simulink model "CanardUAV_Flight_Control_Using_PID"  (R2020b)
settings: Solver=VariableStepAuto  StartTime=0  StopTime=30  FixedStep=1e-4  MaxStep=1e-2  RelTol=1e-3
libraries: slpidlib x6
settings Model: Creator=Adisu  LastModifiedBy=ysDeng
settings DataIOCC: SaveFormat=StructureWithTime  ReturnWorkspaceOutputs=off
settings OptimizationCC: BlockReduction=off  BufferReuse=off
settings DebuggingCC: AlgebraicLoopMsg=none  UnconnectedInputMsg=none  UnconnectedOutputMsg=none  UnconnectedLineMsg=none

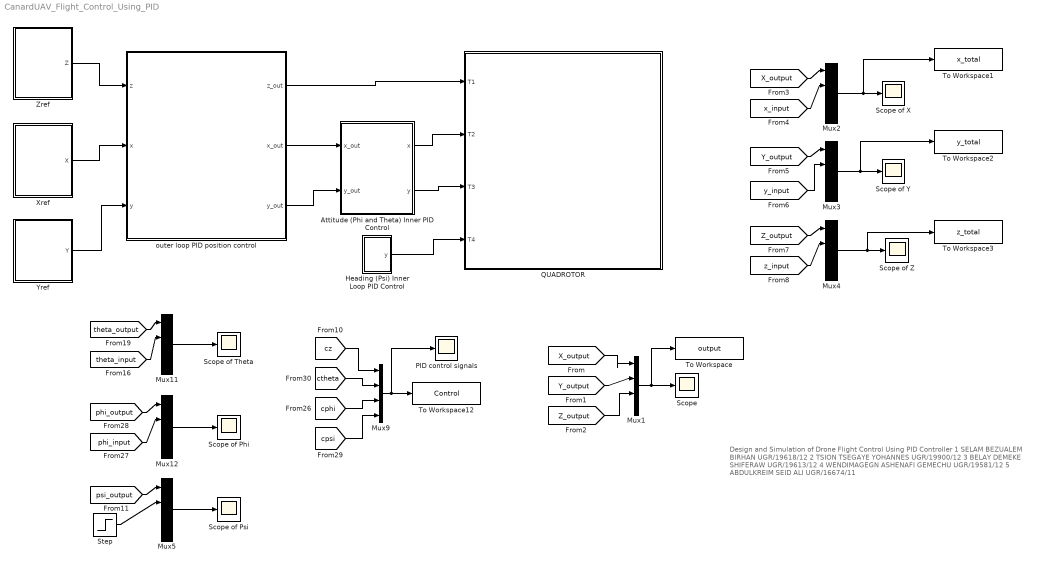
== system CanardUAV_Flight_Control_Using_PID ==
  note: Design and Simulation of Drone Flight Control Using PID Controller
      |
      | 1 SELAM BEZUALEM BIRHAN UGR/19618/12
      | 2 TSION TSEGAYE YOHANNES UGR/19900/12
      | 3 BELAY DEMEKE SHIFERAW UGR/19613/12
      | 4 WENDIMAGEGN ASHENAFI GEMECHU UGR/19581/12
      | 5 ABDULKREIM SEID ALI UGR/16674/11
  Attitude (Phi and Theta) Inner PID Control : Subsystem
  Heading (Psi) Inner Loop PID Control : Subsystem
  Mux1 : Mux  Inputs=3
  Mux{2..5,11..12} (6 alike) : Mux  Inputs=2
  Mux9 : Mux
  PID control signals : Scope
  "QUADROTOR " : Subsystem
      mask Display: image('$imagefile'); % Use "Edit Image" on toolstrip to change.
  Scope : Scope
  Scope of Phi : Scope
  Scope of Psi : Scope
  Scope of Theta : Scope
  Scope of X : Scope
  Scope of Y : Scope
  Scope of Z : Scope
  Step : Step  Time=5  After=0.2  SampleTime=0
  To Workspace : ToWorkspace  VariableName=output  SaveFormat=Timeseries  SampleTime=-1
  To Workspace1 : ToWorkspace  VariableName=x_total  SaveFormat=Timeseries  SampleTime=-1
  To Workspace12 : ToWorkspace  VariableName=Control  SampleTime=-1
      settings: Save2DSignal=2-D array (concatenate along first dimension)
  To Workspace2 : ToWorkspace  VariableName=y_total  SaveFormat=Timeseries  SampleTime=-1
  To Workspace3 : ToWorkspace  VariableName=z_total  SaveFormat=Timeseries  SampleTime=-1
  Xref : Subsystem
      mask Display: image('C:\Users\Mo\Desktop\Porject files\Mathlab\9KgUe.png'); % Use "Edit Image" on toolstrip to change.
  Yref : Subsystem
      mask Display: image('$imagefile'); % Use "Edit Image" on toolstrip to change.
  Zref : Subsystem
      mask Display: image('C:\Users\Mo\Desktop\Porject files\Mathlab\9KgUe.png'); % Use "Edit Image" on toolstrip to change.
  outer loop PID position control : Subsystem
  wires:
  Attitude (Phi and Theta) Inner PID Control/2(y) -> "QUADROTOR "/3(T3)
  outer loop PID position control/3(y_out) -> Attitude (Phi and Theta) Inner PID Control/2(y_out)
  outer loop PID position control/2(x_out) -> Attitude (Phi and Theta) Inner PID Control/1(x_out)
  outer loop PID position control/1(z_out) -> "QUADROTOR "/1(T1)
  Heading (Psi) Inner Loop PID Control/1(y) -> "QUADROTOR "/4(T4)
  Attitude (Phi and Theta) Inner PID Control/1(x) -> "QUADROTOR "/2(T2)
  [theta_input] -> Mux11/2
  Mux11/1 -> Scope of Theta/1
  [theta_output] -> Mux11/1
  [phi_input] -> Mux12/2
  Mux12/1 -> Scope of Phi/1
  [phi_output] -> Mux12/1
  Mux9/1 -> PID control signals/1, To Workspace12/1
  [cz] -> Mux9/1
  Zref/1(Z) -> outer loop PID position control/1(z)
  Xref/1(X) -> outer loop PID position control/2(x)
  Yref/1(Y) -> outer loop PID position control/3(y)
  [X_output] -> Mux1/1
  [Y_output] -> Mux1/2
  [Z_output] -> Mux1/3
  Mux1/1 -> To Workspace/1, Scope/1
  [X_output] -> Mux2/1
  [x_input] -> Mux2/2
  Mux2/1 -> To Workspace1/1, Scope of X/1
  Mux3/1 -> To Workspace2/1, Scope of Y/1
  [y_input] -> Mux3/2
  [Y_output] -> Mux3/1
  [Z_output] -> Mux4/1
  [z_input] -> Mux4/2
  Mux4/1 -> To Workspace3/1, Scope of Z/1
  [psi_output] -> Mux5/1
  Mux5/1 -> Scope of Psi/1
  Step/1 -> Mux5/2
  [ctheta] -> Mux9/2
  [cphi] -> Mux9/3
  [cpsi] -> Mux9/4

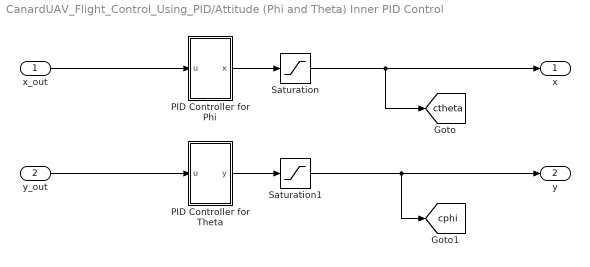
== system CanardUAV_Flight_Control_Using_PID/Attitude (Phi and Theta) Inner PID Control ==
  x_out : Inport
  y_out : Inport  Port=2
  PID Controller for Phi : Subsystem
  PID Controller for Theta : Subsystem
  Saturation : Saturate  UpperLimit=1  LowerLimit=-1
  Saturation1 : Saturate  UpperLimit=1  LowerLimit=-1
  x : Outport
  y : Outport  Port=2
  tag scope: cphi=global, ctheta=global
  wires:
  PID Controller for Phi/1(x) -> Saturation/1
  x_out/1 -> PID Controller for Phi/1(u)
  PID Controller for Theta/1(y) -> Saturation1/1
  Saturation1/1 -> [cphi], y/1
  Saturation/1 -> x/1, [ctheta]
  y_out/1 -> PID Controller for Theta/1(u)

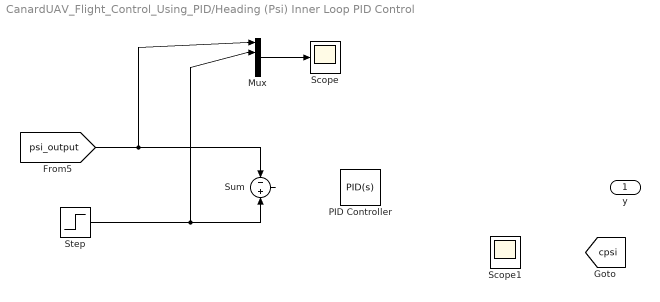
== system CanardUAV_Flight_Control_Using_PID/Heading (Psi) Inner Loop PID Control ==
  Mux : Mux  Inputs=2
  PID Controller : slpidlib/PID Controller  Controller=PID  Form=Parallel  TimeDomain=Continuous-time  UseExternalTs=off  SampleTime=-1  IntegratorMethod=Forward Euler  FilterMethod=Forward Euler  ControllerParametersSource=internal  P=0.000984100095340088  I=4.60704277684503e-05  UseKiTs=off  D=0.00516178120248641  N=5.45397025421619  UseFilter=on  TunerSelectOption=Transfer Function Based (PID Tuner App)  InitialConditionSource=internal  InitialConditionForIntegrator=0  InitialConditionForFilter=0  DifferentiatorICPrevScaledInput=0  ExternalReset=none  TrackingMode=off  Kt=1  LimitOutput=off  SatLimitsSource=internal  UpperSaturationLimit=inf  LowerSaturationLimit=-inf  LinearizeAsGain=on  AntiWindupMode=none  Kb=1  LimitIntegrator=off  UpperIntegratorSaturationLimit=inf  LowerIntegratorSaturationLimit=-inf  POutMin=[]  POutMax=[]  IOutMin=[]  IOutMax=[]  DOutMin=[]  DOutMax=[]  NOutMin=[]  NOutMax=[]  SumOutMin=[]  SumOutMax=[]  SaturationOutMin=[]  SaturationOutMax=[]  PParamMin=[]  PParamMax=[]  IParamMin=[]  IParamMax=[]  DParamMin=[]  DParamMax=[]  NParamMin=[]  NParamMax=[]  KbParamMin=[]  KbParamMax=[]  KtParamMin=[]  KtParamMax=[]  KbOutMin=[]  KbOutMax=[]  KtOutMin=[]  KtOutMax=[]  IntegratorOutMin=[]  IntegratorOutMax=[]  FilterOutMin=[]  FilterOutMax=[]  SumI1OutMin=[]  SumI1OutMax=[]  SumI2OutMin=[]  SumI2OutMax=[]  SumI3OutMin=[]  SumI3OutMax=[]  SumI4OutMin=[]  SumI4OutMax=[]  SumDOutMin=[]  SumDOutMax=[]  DifferentiatorOutMin=[]  DifferentiatorOutMax=[]  FilterDiffOutCoefMin=[]  FilterDiffOutCoefMax=[]  ReciprocalOutMin=[]  ReciprocalOutMax=[]  SumDenOutMin=[]  SumDenOutMax=[]  SumNumOutMin=[]  SumNumOutMax=[]  DivideOutMin=[]  DivideOutMax=[]  UdiffTsProdOutMin=[]  UdiffTsProdOutMax=[]  NTsProdOutMin=[]  NTsProdOutMax=[]  UintegralTsProdOutMin=[]  UintegralTsProdOutMax=[]  UngainTsProdOutMin=[]  UngainTsProdOutMax=[]  ClampingZeroOutDataTypeStr=Inherit: Inherit via back propagation  ClampingZeroOutMin=[]  ClampingZeroOutMax=[]  FilterDenConstantOutDataTypeStr=Inherit: Inherit via back propagation  FilterDenConstantOutMin=[]  FilterDenConstantOutMax=[]  PCopyOutDataTypeStr=Inherit: Inherit via back propagation  PCopyOutMin=[]  PCopyOutMax=[]  NCopyOutDataTypeStr=Inherit: Inherit via back propagation  NCopyOutMin=[]  NCopyOutMax=[]  IntegratorContinuousStateAttributes=''  IntegratorStateMustResolveToSignalObject=off  IntegratorRTWStateStorageClass=Auto  FilterContinuousStateAttributes=''  FilterStateMustResolveToSignalObject=off  FilterRTWStateStorageClass=Auto  ParallelPVariant=InternalParameters  IdealPVariant=Disabled  IVariant=InternalParameters  DVariant=InternalParameters  IntegratorVariant=Continuous  SatVariant=Disabled  AWVariant=Passthrough  PCopyVariant=Disabled  TRVariant=Disabled  FdbkBlocksVariant=Forward  IdealPFdbkVariant=Disabled  SatFdbkVariant=Disabled  DerivativeFilterVariant=ContFilter  NVariant=InternalParameters  NCopyVariant=Disabled  FilterICVariant=InternalICsFilter  IntegratorICVariant=InternalICs  ExternalResetVariant=Disabled  TRSumVariant=Passthrough  SumFdbkVariant=Disabled  SumVariant=Sum_PID  TsampFilterVariant=InternalTs  TsampNgainVariant=Passthrough  TsampIntegralVariant=Disabled_SignalSpec  ExternalSaturationOutDataTypeStr=Inherit: Same as second input
  Scope : Scope
  Scope1 : Scope
  Step : Step  Time=5  After=0.2  SampleTime=0
  Sum : Sum  Inputs=-+
  y : Outport
  tag scope: cpsi=global
  wires:
  [psi_output] -> Mux/1, Sum/1
  Sum/1 -> ?
  Mux/1 -> Scope/1
  ? -> y/1, [cpsi], Scope1/1
  Step/1 -> Sum/2, Mux/2

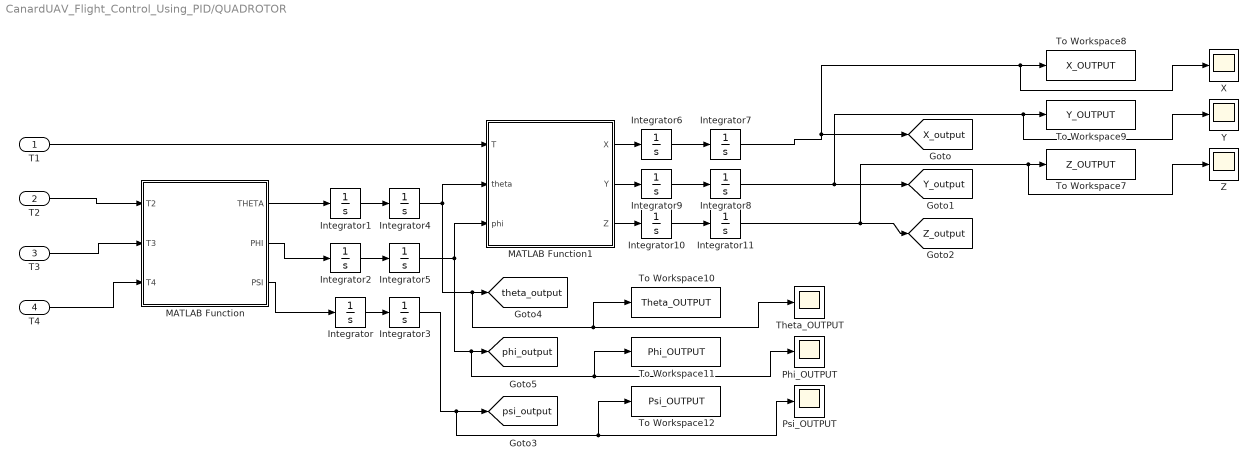
== system CanardUAV_Flight_Control_Using_PID/QUADROTOR  ==
  T1 : Inport
  T2 : Inport  Port=2
  T3 : Inport  Port=3
  T4 : Inport  Port=4
  Integrator{,1..11} (12 alike) : Integrator
  MATLAB Function : MATLAB Function  TreatAsAtomicUnit=on
  MATLAB Function1 : MATLAB Function  TreatAsAtomicUnit=on
  Phi_OUTPUT : Scope
  Psi_OUTPUT : Scope
  Theta_OUTPUT : Scope
  To Workspace10 : ToWorkspace  VariableName=Theta_OUTPUT  SampleTime=-1
      settings: Save2DSignal=2-D array (concatenate along first dimension)
  To Workspace11 : ToWorkspace  VariableName=Phi_OUTPUT  SampleTime=-1
      settings: Save2DSignal=2-D array (concatenate along first dimension)
  To Workspace12 : ToWorkspace  VariableName=Psi_OUTPUT  SampleTime=-1
      settings: Save2DSignal=2-D array (concatenate along first dimension)
  To Workspace7 : ToWorkspace  VariableName=Z_OUTPUT  SampleTime=-1
      settings: Save2DSignal=2-D array (concatenate along first dimension)
  To Workspace8 : ToWorkspace  VariableName=X_OUTPUT  SampleTime=-1
      settings: Save2DSignal=2-D array (concatenate along first dimension)
  To Workspace9 : ToWorkspace  VariableName=Y_OUTPUT  SampleTime=-1
      settings: Save2DSignal=2-D array (concatenate along first dimension)
  X : Scope
  Y : Scope
  Z : Scope
  tag scope: X_output=global, Y_output=global, Z_output=global, phi_output=global, psi_output=global, theta_output=global
  wires:
  MATLAB Function/3(PSI) -> Integrator/1
  Integrator9/1 -> Integrator8/1
  Integrator10/1 -> Integrator11/1
  Integrator6/1 -> Integrator7/1
  Integrator1/1 -> Integrator4/1
  MATLAB Function1/2(Y) -> Integrator9/1
  Integrator2/1 -> Integrator5/1
  MATLAB Function1/1(X) -> Integrator6/1
  MATLAB Function1/3(Z) -> Integrator10/1
  Integrator/1 -> Integrator3/1
  MATLAB Function/1(THETA) -> Integrator1/1
  T2/1 -> MATLAB Function/1(T2)
  MATLAB Function/2(PHI) -> Integrator2/1
  Integrator8/1 -> Y/1, To Workspace9/1, [Y_output]
  Integrator4/1 -> To Workspace10/1, Theta_OUTPUT/1, [theta_output], MATLAB Function1/2(theta)
  T1/1 -> MATLAB Function1/1(T)
  Integrator5/1 -> To Workspace11/1, Phi_OUTPUT/1, [phi_output], MATLAB Function1/3(phi)
  T3/1 -> MATLAB Function/2(T3)
  Integrator11/1 -> Z/1, To Workspace7/1, [Z_output]
  T4/1 -> MATLAB Function/3(T4)
  Integrator3/1 -> Psi_OUTPUT/1, To Workspace12/1, [psi_output]
  Integrator7/1 -> X/1, To Workspace8/1, [X_output]

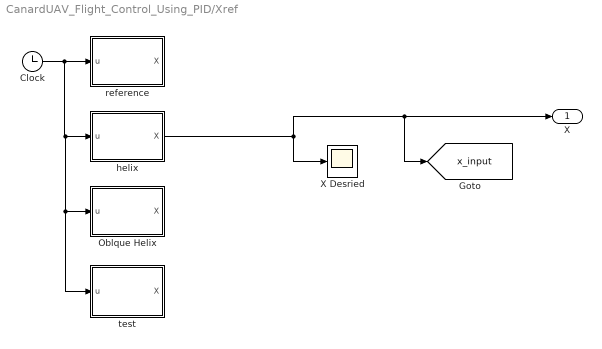
== system CanardUAV_Flight_Control_Using_PID/Xref ==
  Clock : Clock
      settings: Decimation=200
  Oblque Helix : MATLAB Function  TreatAsAtomicUnit=on
  X Desried : Scope
  helix : MATLAB Function  TreatAsAtomicUnit=on
  reference : MATLAB Function  TreatAsAtomicUnit=on
  test : MATLAB Function  TreatAsAtomicUnit=on
  X : Outport
  tag scope: x_input=global
  wires:
  helix/1(X) -> X Desried/1, [x_input], X/1
  Clock/1 -> test/1(u), Oblque Helix/1(u), helix/1(u), reference/1(u)

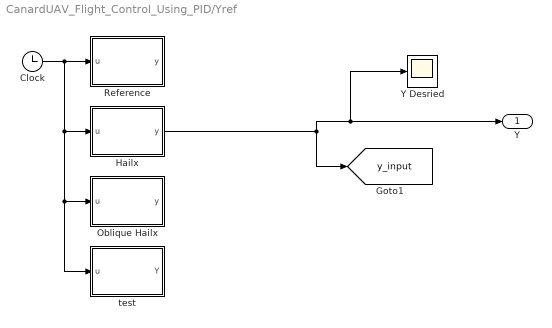
== system CanardUAV_Flight_Control_Using_PID/Yref ==
  Clock : Clock
      settings: Decimation=200
  Hailx : MATLAB Function  TreatAsAtomicUnit=on
  Oblique Hailx : MATLAB Function  TreatAsAtomicUnit=on
  Reference : MATLAB Function  TreatAsAtomicUnit=on
  Y Desried : Scope
  test : MATLAB Function  TreatAsAtomicUnit=on
  Y : Outport
  tag scope: y_input=global
  wires:
  Hailx/1(y) -> [y_input], Y Desried/1, Y/1
  Clock/1 -> test/1(u), Oblique Hailx/1(u), Hailx/1(u), Reference/1(u)

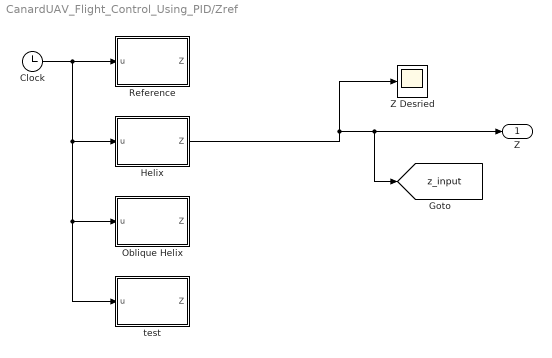
== system CanardUAV_Flight_Control_Using_PID/Zref ==
  Clock : Clock
      settings: Decimation=200
  Helix : MATLAB Function  TreatAsAtomicUnit=on
  Oblique Helix : MATLAB Function  TreatAsAtomicUnit=on
  Reference : MATLAB Function  TreatAsAtomicUnit=on
  Z Desried : Scope
  test : MATLAB Function  TreatAsAtomicUnit=on
  Z : Outport
  tag scope: z_input=global
  wires:
  Helix/1(Z) -> Z Desried/1, [z_input], Z/1
  Clock/1 -> Reference/1(u), Helix/1(u), test/1(u), Oblique Helix/1(u)

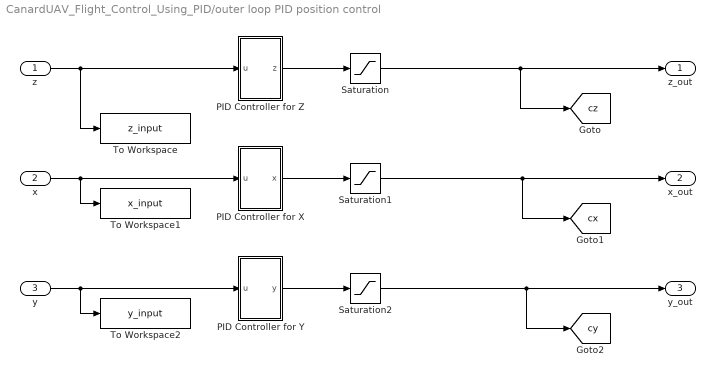
== system CanardUAV_Flight_Control_Using_PID/outer loop PID position control ==
  z : Inport
  x : Inport  Port=2
  y : Inport  Port=3
  PID Controller for X : Subsystem
  PID Controller for Y : Subsystem
  PID Controller for Z : Subsystem
  Saturation : Saturate  UpperLimit=8  LowerLimit=0
  Saturation1 : Saturate  UpperLimit=1  LowerLimit=-1
  Saturation2 : Saturate  UpperLimit=1  LowerLimit=-1
  To Workspace : ToWorkspace  VariableName=z_input  SaveFormat=Timeseries  SampleTime=-1
  To Workspace1 : ToWorkspace  VariableName=x_input  SaveFormat=Timeseries  SampleTime=-1
  To Workspace2 : ToWorkspace  VariableName=y_input  SaveFormat=Timeseries  SampleTime=-1
  z_out : Outport
  x_out : Outport  Port=2
  y_out : Outport  Port=3
  tag scope: cx=global, cy=global, cz=global
  wires:
  PID Controller for Z/1(z) -> Saturation/1
  PID Controller for Y/1(y) -> Saturation2/1
  PID Controller for X/1(x) -> Saturation1/1
  z/1 -> To Workspace/1, PID Controller for Z/1(u)
  Saturation/1 -> [cz], z_out/1
  Saturation1/1 -> x_out/1, [cx]
  Saturation2/1 -> y_out/1, [cy]
  x/1 -> To Workspace1/1, PID Controller for X/1(u)
  y/1 -> To Workspace2/1, PID Controller for Y/1(u)

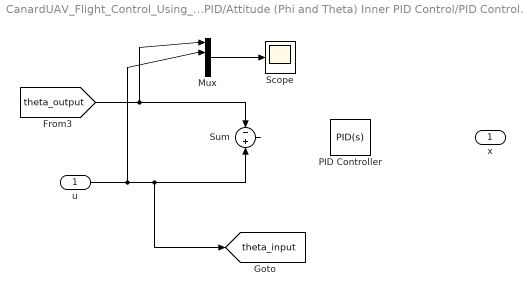
== system CanardUAV_Flight_Control_Using_PID/Attitude (Phi and Theta) Inner PID Control/PID Controller for Phi ==
  u : Inport
  Mux : Mux  Inputs=2
  PID Controller : slpidlib/PID Controller  Controller=PID  Form=Parallel  TimeDomain=Continuous-time  UseExternalTs=off  SampleTime=-1  IntegratorMethod=Forward Euler  FilterMethod=Forward Euler  ControllerParametersSource=internal  P=1.9891252123158  I=5.9601995006883  UseKiTs=off  D=0.159826669701916  N=399.033800628707  UseFilter=on  TunerSelectOption=Transfer Function Based (PID Tuner App)  InitialConditionSource=internal  InitialConditionForIntegrator=0  InitialConditionForFilter=0  DifferentiatorICPrevScaledInput=0  ExternalReset=none  TrackingMode=off  Kt=1  LimitOutput=off  SatLimitsSource=internal  UpperSaturationLimit=inf  LowerSaturationLimit=-inf  LinearizeAsGain=on  AntiWindupMode=none  Kb=1  LimitIntegrator=off  UpperIntegratorSaturationLimit=inf  LowerIntegratorSaturationLimit=-inf  POutMin=[]  POutMax=[]  IOutMin=[]  IOutMax=[]  DOutMin=[]  DOutMax=[]  NOutMin=[]  NOutMax=[]  SumOutMin=[]  SumOutMax=[]  SaturationOutMin=[]  SaturationOutMax=[]  PParamMin=[]  PParamMax=[]  IParamMin=[]  IParamMax=[]  DParamMin=[]  DParamMax=[]  NParamMin=[]  NParamMax=[]  KbParamMin=[]  KbParamMax=[]  KtParamMin=[]  KtParamMax=[]  KbOutMin=[]  KbOutMax=[]  KtOutMin=[]  KtOutMax=[]  IntegratorOutMin=[]  IntegratorOutMax=[]  FilterOutMin=[]  FilterOutMax=[]  SumI1OutMin=[]  SumI1OutMax=[]  SumI2OutMin=[]  SumI2OutMax=[]  SumI3OutMin=[]  SumI3OutMax=[]  SumI4OutMin=[]  SumI4OutMax=[]  SumDOutMin=[]  SumDOutMax=[]  DifferentiatorOutMin=[]  DifferentiatorOutMax=[]  FilterDiffOutCoefMin=[]  FilterDiffOutCoefMax=[]  ReciprocalOutMin=[]  ReciprocalOutMax=[]  SumDenOutMin=[]  SumDenOutMax=[]  SumNumOutMin=[]  SumNumOutMax=[]  DivideOutMin=[]  DivideOutMax=[]  UdiffTsProdOutMin=[]  UdiffTsProdOutMax=[]  NTsProdOutMin=[]  NTsProdOutMax=[]  UintegralTsProdOutMin=[]  UintegralTsProdOutMax=[]  UngainTsProdOutMin=[]  UngainTsProdOutMax=[]  ClampingZeroOutDataTypeStr=Inherit: Inherit via back propagation  ClampingZeroOutMin=[]  ClampingZeroOutMax=[]  FilterDenConstantOutDataTypeStr=Inherit: Inherit via back propagation  FilterDenConstantOutMin=[]  FilterDenConstantOutMax=[]  PCopyOutDataTypeStr=Inherit: Inherit via back propagation  PCopyOutMin=[]  PCopyOutMax=[]  NCopyOutDataTypeStr=Inherit: Inherit via back propagation  NCopyOutMin=[]  NCopyOutMax=[]  IntegratorContinuousStateAttributes=''  IntegratorStateMustResolveToSignalObject=off  IntegratorRTWStateStorageClass=Auto  FilterContinuousStateAttributes=''  FilterStateMustResolveToSignalObject=off  FilterRTWStateStorageClass=Auto  ParallelPVariant=InternalParameters  IdealPVariant=Disabled  IVariant=InternalParameters  DVariant=InternalParameters  IntegratorVariant=Continuous  SatVariant=Disabled  AWVariant=Passthrough  PCopyVariant=Disabled  TRVariant=Disabled  FdbkBlocksVariant=Forward  IdealPFdbkVariant=Disabled  SatFdbkVariant=Disabled  DerivativeFilterVariant=ContFilter  NVariant=InternalParameters  NCopyVariant=Disabled  FilterICVariant=InternalICsFilter  IntegratorICVariant=InternalICs  ExternalResetVariant=Disabled  TRSumVariant=Passthrough  SumFdbkVariant=Disabled  SumVariant=Sum_PID  TsampFilterVariant=InternalTs  TsampNgainVariant=Passthrough  TsampIntegralVariant=Disabled_SignalSpec  ExternalSaturationOutDataTypeStr=Inherit: Same as second input
  Scope : Scope
  Sum : Sum  Inputs=-+
  x : Outport
  tag scope: theta_input=global
  wires:
  [theta_output] -> Mux/1, Sum/1
  u/1 -> Mux/2, [theta_input], Sum/2
  Sum/1 -> ?
  Mux/1 -> Scope/1
  ? -> x/1

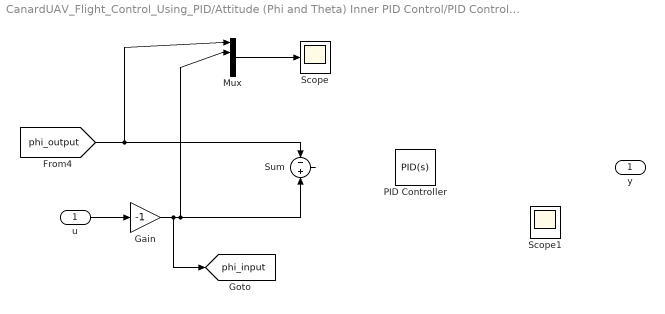
== system CanardUAV_Flight_Control_Using_PID/Attitude (Phi and Theta) Inner PID Control/PID Controller for Theta ==
  u : Inport
  Gain : Gain  Gain=-1
  Mux : Mux  Inputs=2
  PID Controller : slpidlib/PID Controller  Controller=PID  Form=Parallel  TimeDomain=Continuous-time  UseExternalTs=off  SampleTime=-1  IntegratorMethod=Forward Euler  FilterMethod=Forward Euler  ControllerParametersSource=internal  P=0.0999  I=0.01  UseKiTs=off  D=0.22  N=100  UseFilter=on  TunerSelectOption=Transfer Function Based (PID Tuner App)  InitialConditionSource=internal  InitialConditionForIntegrator=0  InitialConditionForFilter=0  DifferentiatorICPrevScaledInput=0  ExternalReset=none  TrackingMode=off  Kt=1  LimitOutput=off  SatLimitsSource=internal  UpperSaturationLimit=inf  LowerSaturationLimit=-inf  LinearizeAsGain=on  AntiWindupMode=none  Kb=1  LimitIntegrator=off  UpperIntegratorSaturationLimit=inf  LowerIntegratorSaturationLimit=-inf  POutMin=[]  POutMax=[]  IOutMin=[]  IOutMax=[]  DOutMin=[]  DOutMax=[]  NOutMin=[]  NOutMax=[]  SumOutMin=[]  SumOutMax=[]  SaturationOutMin=[]  SaturationOutMax=[]  PParamMin=[]  PParamMax=[]  IParamMin=[]  IParamMax=[]  DParamMin=[]  DParamMax=[]  NParamMin=[]  NParamMax=[]  KbParamMin=[]  KbParamMax=[]  KtParamMin=[]  KtParamMax=[]  KbOutMin=[]  KbOutMax=[]  KtOutMin=[]  KtOutMax=[]  IntegratorOutMin=[]  IntegratorOutMax=[]  FilterOutMin=[]  FilterOutMax=[]  SumI1OutMin=[]  SumI1OutMax=[]  SumI2OutMin=[]  SumI2OutMax=[]  SumI3OutMin=[]  SumI3OutMax=[]  SumI4OutMin=[]  SumI4OutMax=[]  SumDOutMin=[]  SumDOutMax=[]  DifferentiatorOutMin=[]  DifferentiatorOutMax=[]  FilterDiffOutCoefMin=[]  FilterDiffOutCoefMax=[]  ReciprocalOutMin=[]  ReciprocalOutMax=[]  SumDenOutMin=[]  SumDenOutMax=[]  SumNumOutMin=[]  SumNumOutMax=[]  DivideOutMin=[]  DivideOutMax=[]  UdiffTsProdOutMin=[]  UdiffTsProdOutMax=[]  NTsProdOutMin=[]  NTsProdOutMax=[]  UintegralTsProdOutMin=[]  UintegralTsProdOutMax=[]  UngainTsProdOutMin=[]  UngainTsProdOutMax=[]  ClampingZeroOutDataTypeStr=Inherit: Inherit via back propagation  ClampingZeroOutMin=[]  ClampingZeroOutMax=[]  FilterDenConstantOutDataTypeStr=Inherit: Inherit via back propagation  FilterDenConstantOutMin=[]  FilterDenConstantOutMax=[]  PCopyOutDataTypeStr=Inherit: Inherit via back propagation  PCopyOutMin=[]  PCopyOutMax=[]  NCopyOutDataTypeStr=Inherit: Inherit via back propagation  NCopyOutMin=[]  NCopyOutMax=[]  IntegratorContinuousStateAttributes=''  IntegratorStateMustResolveToSignalObject=off  IntegratorRTWStateStorageClass=Auto  FilterContinuousStateAttributes=''  FilterStateMustResolveToSignalObject=off  FilterRTWStateStorageClass=Auto  ParallelPVariant=InternalParameters  IdealPVariant=Disabled  IVariant=InternalParameters  DVariant=InternalParameters  IntegratorVariant=Continuous  SatVariant=Disabled  AWVariant=Passthrough  PCopyVariant=Disabled  TRVariant=Disabled  FdbkBlocksVariant=Forward  IdealPFdbkVariant=Disabled  SatFdbkVariant=Disabled  DerivativeFilterVariant=ContFilter  NVariant=InternalParameters  NCopyVariant=Disabled  FilterICVariant=InternalICsFilter  IntegratorICVariant=InternalICs  ExternalResetVariant=Disabled  TRSumVariant=Passthrough  SumFdbkVariant=Disabled  SumVariant=Sum_PID  TsampFilterVariant=InternalTs  TsampNgainVariant=Passthrough  TsampIntegralVariant=Disabled_SignalSpec  ExternalSaturationOutDataTypeStr=Inherit: Same as second input
  Scope : Scope
  Scope1 : Scope
  Sum : Sum  Inputs=-+
  y : Outport
  tag scope: phi_input=global
  wires:
  [phi_output] -> Mux/1, Sum/1
  Mux/1 -> Scope/1
  Sum/1 -> ?
  u/1 -> Gain/1
  Gain/1 -> [phi_input], Mux/2, Sum/2
  ? -> y/1, Scope1/1

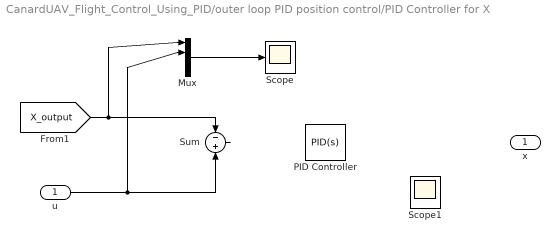
== system CanardUAV_Flight_Control_Using_PID/outer loop PID position control/PID Controller for X ==
  u : Inport
  Mux : Mux  Inputs=2
  PID Controller : slpidlib/PID Controller  Controller=PID  Form=Parallel  TimeDomain=Continuous-time  UseExternalTs=off  SampleTime=-1  IntegratorMethod=Forward Euler  FilterMethod=Forward Euler  ControllerParametersSource=internal  P=0.0999  I=0.031  UseKiTs=off  D=0.22  N=100  UseFilter=on  TunerSelectOption=Transfer Function Based (PID Tuner App)  InitialConditionSource=internal  InitialConditionForIntegrator=0  InitialConditionForFilter=0  DifferentiatorICPrevScaledInput=0  ExternalReset=none  TrackingMode=off  Kt=1  LimitOutput=off  SatLimitsSource=internal  UpperSaturationLimit=inf  LowerSaturationLimit=-inf  LinearizeAsGain=on  AntiWindupMode=none  Kb=1  LimitIntegrator=off  UpperIntegratorSaturationLimit=inf  LowerIntegratorSaturationLimit=-inf  POutMin=[]  POutMax=[]  IOutMin=[]  IOutMax=[]  DOutMin=[]  DOutMax=[]  NOutMin=[]  NOutMax=[]  SumOutMin=[]  SumOutMax=[]  SaturationOutMin=[]  SaturationOutMax=[]  PParamMin=[]  PParamMax=[]  IParamMin=[]  IParamMax=[]  DParamMin=[]  DParamMax=[]  NParamMin=[]  NParamMax=[]  KbParamMin=[]  KbParamMax=[]  KtParamMin=[]  KtParamMax=[]  KbOutMin=[]  KbOutMax=[]  KtOutMin=[]  KtOutMax=[]  IntegratorOutMin=[]  IntegratorOutMax=[]  FilterOutMin=[]  FilterOutMax=[]  SumI1OutMin=[]  SumI1OutMax=[]  SumI2OutMin=[]  SumI2OutMax=[]  SumI3OutMin=[]  SumI3OutMax=[]  SumI4OutMin=[]  SumI4OutMax=[]  SumDOutMin=[]  SumDOutMax=[]  DifferentiatorOutMin=[]  DifferentiatorOutMax=[]  FilterDiffOutCoefMin=[]  FilterDiffOutCoefMax=[]  ReciprocalOutMin=[]  ReciprocalOutMax=[]  SumDenOutMin=[]  SumDenOutMax=[]  SumNumOutMin=[]  SumNumOutMax=[]  DivideOutMin=[]  DivideOutMax=[]  UdiffTsProdOutMin=[]  UdiffTsProdOutMax=[]  NTsProdOutMin=[]  NTsProdOutMax=[]  UintegralTsProdOutMin=[]  UintegralTsProdOutMax=[]  UngainTsProdOutMin=[]  UngainTsProdOutMax=[]  ClampingZeroOutDataTypeStr=Inherit: Inherit via back propagation  ClampingZeroOutMin=[]  ClampingZeroOutMax=[]  FilterDenConstantOutDataTypeStr=Inherit: Inherit via back propagation  FilterDenConstantOutMin=[]  FilterDenConstantOutMax=[]  PCopyOutDataTypeStr=Inherit: Inherit via back propagation  PCopyOutMin=[]  PCopyOutMax=[]  NCopyOutDataTypeStr=Inherit: Inherit via back propagation  NCopyOutMin=[]  NCopyOutMax=[]  IntegratorContinuousStateAttributes=''  IntegratorStateMustResolveToSignalObject=off  IntegratorRTWStateStorageClass=Auto  FilterContinuousStateAttributes=''  FilterStateMustResolveToSignalObject=off  FilterRTWStateStorageClass=Auto  ParallelPVariant=InternalParameters  IdealPVariant=Disabled  IVariant=InternalParameters  DVariant=InternalParameters  IntegratorVariant=Continuous  SatVariant=Disabled  AWVariant=Passthrough  PCopyVariant=Disabled  TRVariant=Disabled  FdbkBlocksVariant=Forward  IdealPFdbkVariant=Disabled  SatFdbkVariant=Disabled  DerivativeFilterVariant=ContFilter  NVariant=InternalParameters  NCopyVariant=Disabled  FilterICVariant=InternalICsFilter  IntegratorICVariant=InternalICs  ExternalResetVariant=Disabled  TRSumVariant=Passthrough  SumFdbkVariant=Disabled  SumVariant=Sum_PID  TsampFilterVariant=InternalTs  TsampNgainVariant=Passthrough  TsampIntegralVariant=Disabled_SignalSpec  ExternalSaturationOutDataTypeStr=Inherit: Same as second input
  Scope : Scope
  Scope1 : Scope
  Sum : Sum  Inputs=-+
  x : Outport
  wires:
  [X_output] -> Mux/1, Sum/1
  u/1 -> Mux/2, Sum/2
  Sum/1 -> ?
  Mux/1 -> Scope/1
  ? -> x/1, Scope1/1

== system CanardUAV_Flight_Control_Using_PID/outer loop PID position control/PID Controller for Y ==
  u : Inport
  Mux : Mux  Inputs=2
  PID Controller : slpidlib/PID Controller  Controller=PID  Form=Parallel  TimeDomain=Continuous-time  UseExternalTs=off  SampleTime=-1  IntegratorMethod=Forward Euler  FilterMethod=Forward Euler  ControllerParametersSource=internal  P=4.84190302545016  I=1.13406263808077  UseKiTs=off  D=3.19909563995476  N=3783.08190114897  UseFilter=on  TunerSelectOption=Transfer Function Based (PID Tuner App)  InitialConditionSource=internal  InitialConditionForIntegrator=0  InitialConditionForFilter=0  DifferentiatorICPrevScaledInput=0  ExternalReset=none  TrackingMode=off  Kt=1  LimitOutput=off  SatLimitsSource=internal  UpperSaturationLimit=inf  LowerSaturationLimit=-inf  LinearizeAsGain=on  AntiWindupMode=none  Kb=1  LimitIntegrator=off  UpperIntegratorSaturationLimit=inf  LowerIntegratorSaturationLimit=-inf  POutMin=[]  POutMax=[]  IOutMin=[]  IOutMax=[]  DOutMin=[]  DOutMax=[]  NOutMin=[]  NOutMax=[]  SumOutMin=[]  SumOutMax=[]  SaturationOutMin=[]  SaturationOutMax=[]  PParamMin=[]  PParamMax=[]  IParamMin=[]  IParamMax=[]  DParamMin=[]  DParamMax=[]  NParamMin=[]  NParamMax=[]  KbParamMin=[]  KbParamMax=[]  KtParamMin=[]  KtParamMax=[]  KbOutMin=[]  KbOutMax=[]  KtOutMin=[]  KtOutMax=[]  IntegratorOutMin=[]  IntegratorOutMax=[]  FilterOutMin=[]  FilterOutMax=[]  SumI1OutMin=[]  SumI1OutMax=[]  SumI2OutMin=[]  SumI2OutMax=[]  SumI3OutMin=[]  SumI3OutMax=[]  SumI4OutMin=[]  SumI4OutMax=[]  SumDOutMin=[]  SumDOutMax=[]  DifferentiatorOutMin=[]  DifferentiatorOutMax=[]  FilterDiffOutCoefMin=[]  FilterDiffOutCoefMax=[]  ReciprocalOutMin=[]  ReciprocalOutMax=[]  SumDenOutMin=[]  SumDenOutMax=[]  SumNumOutMin=[]  SumNumOutMax=[]  DivideOutMin=[]  DivideOutMax=[]  UdiffTsProdOutMin=[]  UdiffTsProdOutMax=[]  NTsProdOutMin=[]  NTsProdOutMax=[]  UintegralTsProdOutMin=[]  UintegralTsProdOutMax=[]  UngainTsProdOutMin=[]  UngainTsProdOutMax=[]  ClampingZeroOutDataTypeStr=Inherit: Inherit via back propagation  ClampingZeroOutMin=[]  ClampingZeroOutMax=[]  FilterDenConstantOutDataTypeStr=Inherit: Inherit via back propagation  FilterDenConstantOutMin=[]  FilterDenConstantOutMax=[]  PCopyOutDataTypeStr=Inherit: Inherit via back propagation  PCopyOutMin=[]  PCopyOutMax=[]  NCopyOutDataTypeStr=Inherit: Inherit via back propagation  NCopyOutMin=[]  NCopyOutMax=[]  IntegratorContinuousStateAttributes=''  IntegratorStateMustResolveToSignalObject=off  IntegratorRTWStateStorageClass=Auto  FilterContinuousStateAttributes=''  FilterStateMustResolveToSignalObject=off  FilterRTWStateStorageClass=Auto  ParallelPVariant=InternalParameters  IdealPVariant=Disabled  IVariant=InternalParameters  DVariant=InternalParameters  IntegratorVariant=Continuous  SatVariant=Disabled  AWVariant=Passthrough  PCopyVariant=Disabled  TRVariant=Disabled  FdbkBlocksVariant=Forward  IdealPFdbkVariant=Disabled  SatFdbkVariant=Disabled  DerivativeFilterVariant=ContFilter  NVariant=InternalParameters  NCopyVariant=Disabled  FilterICVariant=InternalICsFilter  IntegratorICVariant=InternalICs  ExternalResetVariant=Disabled  TRSumVariant=Passthrough  SumFdbkVariant=Disabled  SumVariant=Sum_PID  TsampFilterVariant=InternalTs  TsampNgainVariant=Passthrough  TsampIntegralVariant=Disabled_SignalSpec  ExternalSaturationOutDataTypeStr=Inherit: Same as second input
  Scope : Scope
  Scope1 : Scope
  Sum : Sum  Inputs=-+
  y : Outport
  wires:
  [Y_output] -> Mux/1, Sum/1
  Sum/1 -> ?
  Mux/1 -> Scope/1
  ? -> y/1, Scope1/1
  u/1 -> Mux/2, Sum/2

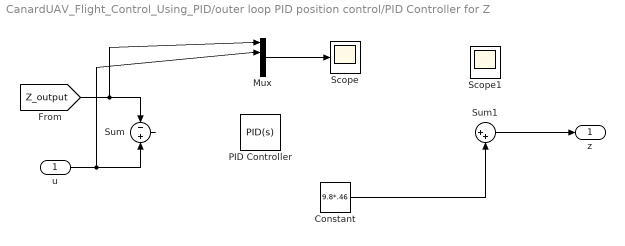
== system CanardUAV_Flight_Control_Using_PID/outer loop PID position control/PID Controller for Z ==
  u : Inport
  Constant : Constant  Value=9.8*.46
  Mux : Mux  Inputs=2
  PID Controller : slpidlib/PID Controller  Controller=PID  Form=Parallel  TimeDomain=Continuous-time  UseExternalTs=off  SampleTime=-1  IntegratorMethod=Forward Euler  FilterMethod=Forward Euler  ControllerParametersSource=internal  P=0.0854124611049774  I=0.00399856542895931  UseKiTs=off  D=0.448003651536497  N=5.45397025421619  UseFilter=on  TunerSelectOption=Transfer Function Based (PID Tuner App)  InitialConditionSource=internal  InitialConditionForIntegrator=0  InitialConditionForFilter=0  DifferentiatorICPrevScaledInput=0  ExternalReset=none  TrackingMode=off  Kt=1  LimitOutput=off  SatLimitsSource=internal  UpperSaturationLimit=inf  LowerSaturationLimit=-inf  LinearizeAsGain=on  AntiWindupMode=none  Kb=1  LimitIntegrator=off  UpperIntegratorSaturationLimit=inf  LowerIntegratorSaturationLimit=-inf  POutMin=[]  POutMax=[]  IOutMin=[]  IOutMax=[]  DOutMin=[]  DOutMax=[]  NOutMin=[]  NOutMax=[]  SumOutMin=[]  SumOutMax=[]  SaturationOutMin=[]  SaturationOutMax=[]  PParamMin=[]  PParamMax=[]  IParamMin=[]  IParamMax=[]  DParamMin=[]  DParamMax=[]  NParamMin=[]  NParamMax=[]  KbParamMin=[]  KbParamMax=[]  KtParamMin=[]  KtParamMax=[]  KbOutMin=[]  KbOutMax=[]  KtOutMin=[]  KtOutMax=[]  IntegratorOutMin=[]  IntegratorOutMax=[]  FilterOutMin=[]  FilterOutMax=[]  SumI1OutMin=[]  SumI1OutMax=[]  SumI2OutMin=[]  SumI2OutMax=[]  SumI3OutMin=[]  SumI3OutMax=[]  SumI4OutMin=[]  SumI4OutMax=[]  SumDOutMin=[]  SumDOutMax=[]  DifferentiatorOutMin=[]  DifferentiatorOutMax=[]  FilterDiffOutCoefMin=[]  FilterDiffOutCoefMax=[]  ReciprocalOutMin=[]  ReciprocalOutMax=[]  SumDenOutMin=[]  SumDenOutMax=[]  SumNumOutMin=[]  SumNumOutMax=[]  DivideOutMin=[]  DivideOutMax=[]  UdiffTsProdOutMin=[]  UdiffTsProdOutMax=[]  NTsProdOutMin=[]  NTsProdOutMax=[]  UintegralTsProdOutMin=[]  UintegralTsProdOutMax=[]  UngainTsProdOutMin=[]  UngainTsProdOutMax=[]  ClampingZeroOutDataTypeStr=Inherit: Inherit via back propagation  ClampingZeroOutMin=[]  ClampingZeroOutMax=[]  FilterDenConstantOutDataTypeStr=Inherit: Inherit via back propagation  FilterDenConstantOutMin=[]  FilterDenConstantOutMax=[]  PCopyOutDataTypeStr=Inherit: Inherit via back propagation  PCopyOutMin=[]  PCopyOutMax=[]  NCopyOutDataTypeStr=Inherit: Inherit via back propagation  NCopyOutMin=[]  NCopyOutMax=[]  IntegratorContinuousStateAttributes=''  IntegratorStateMustResolveToSignalObject=off  IntegratorRTWStateStorageClass=Auto  FilterContinuousStateAttributes=''  FilterStateMustResolveToSignalObject=off  FilterRTWStateStorageClass=Auto  ParallelPVariant=InternalParameters  IdealPVariant=Disabled  IVariant=InternalParameters  DVariant=InternalParameters  IntegratorVariant=Continuous  SatVariant=Disabled  AWVariant=Passthrough  PCopyVariant=Disabled  TRVariant=Disabled  FdbkBlocksVariant=Forward  IdealPFdbkVariant=Disabled  SatFdbkVariant=Disabled  DerivativeFilterVariant=ContFilter  NVariant=InternalParameters  NCopyVariant=Disabled  FilterICVariant=InternalICsFilter  IntegratorICVariant=InternalICs  ExternalResetVariant=Disabled  TRSumVariant=Passthrough  SumFdbkVariant=Disabled  SumVariant=Sum_PID  TsampFilterVariant=InternalTs  TsampNgainVariant=Passthrough  TsampIntegralVariant=Disabled_SignalSpec  ExternalSaturationOutDataTypeStr=Inherit: Same as second input
  Scope : Scope
  Scope1 : Scope
  Sum : Sum  Inputs=-+
  Sum1 : Sum  Inputs=|++
  z : Outport
  wires:
  [Z_output] -> Mux/1, Sum/1
  u/1 -> Mux/2, Sum/2
  Sum/1 -> ?
  Mux/1 -> Scope/1
  Constant/1 -> Sum1/2
  Sum1/1 -> z/1
  ? -> Scope1/1, Sum1/1

== matlab function CanardUAV_Flight_Control_Using_PID/Zref/Helix ==
  data: u input; Z output
function Z = fcn(u)

Z =2+u; %helix

== matlab function CanardUAV_Flight_Control_Using_PID/Yref/Oblique Hailx ==
  data: u input; y output
function y = fcn(u)

y = 5*cos(u); % oblique hailx

== matlab function CanardUAV_Flight_Control_Using_PID/Xref/helix ==
  data: u input; X output
function X = fcn(u)
 
X = sin(u);

== matlab function CanardUAV_Flight_Control_Using_PID/Zref/Oblique Helix ==
  data: u input; Z output
function Z = fcn(u)

Z = u; %oblique helix

== matlab function CanardUAV_Flight_Control_Using_PID/Xref/Oblque Helix ==
  data: u input; X output
function X = fcn(u)

X = 5 + u;

== matlab function CanardUAV_Flight_Control_Using_PID/Yref/Hailx ==
  data: u input; y output
function y = fcn(u)

y = 5*cos(u); % hailx

== matlab function CanardUAV_Flight_Control_Using_PID/Zref/test ==
  data: u input; Z output
function Z = fcn(u)


if u<5
    Z=0;
else
    Z=1;
end

== matlab function CanardUAV_Flight_Control_Using_PID/Xref/test ==
  data: u input; X output
function X = fcn(u)


if u<5
    X=0;
else
    X=1;
end

== matlab function CanardUAV_Flight_Control_Using_PID/Yref/test ==
  data: u input; Y output
function Y = fcn(u)


if u<5
    Y=0;
else
    Y=1;
end

== matlab function CanardUAV_Flight_Control_Using_PID/Yref/Reference ==
  data: u input; y output
function y = fcn(u)
if u>=0&&u<70
y = 0;
elseif u>=70&&u<90 
          y=((-1)/(90-70)*(u-70));   
elseif u>=90&&u<150
               y=-1;
elseif u>=150&&u<170 
          y=(1)/(170-150)*(u-150)-1; 
else 
               y=0;
end

== matlab function CanardUAV_Flight_Control_Using_PID/Xref/reference ==
  data: u input; X output
function X = fcn(u)
if u>=0&&u<30
X = 0;
elseif u>=30&&u<50 
          X=((-1)/(50-30)*(u-30));   
elseif u>=50&&u<70
               X=-1;
elseif u>=70&&u<80 
          X=((-1.5+1)/(80-70)*(u-70))-1;
elseif u>=80&&u<90 
          X=(0.5)/(90-80)*(u-80)-1.5; 
          elseif u>=90&&u<110
               X=-1;
elseif u>=110&&u<130 
          X=(1)/(130-110)*(u-110)-1;
    elseif u>=130&&u<150
               X=0; 
    elseif u>=150&&u<160 
          X=(0.5)/(160-150)*(u-150);
      elseif u>=160&&u<170 
          X=((-0.5)/(170-160)*(u-160))+0.5;    
else 
               X=0;
end

== matlab function CanardUAV_Flight_Control_Using_PID/Zref/Reference ==
  data: u input; Z output
function Z = fcn(u)
if u>=0&&u<15
    Z = 0;
elseif u>=15&&u<55
    Z=0.75;
elseif u>=55&&u<65 
    Z=((1.5-0.75)/(65-55))*(u-55)+0.75;
elseif u>=65&&u<90
    Z=1.5;
elseif u>=90&&u<110 
    Z=((0.75-1.5)/(110-90)*(u-90))+1.5;   
elseif u>=110&&u<135
    Z=0.75;
elseif u>=135&&u<145 
    Z=(1.5-0.75)/(145-135)*(u-135)+0.75;
elseif u>=145&&u<175
    Z=1.5;
elseif u>=175&&u<185 
    Z=((0.75-1.5)/(185-175)*(u-175))+1.5;  
else 
    Z=0.75;
end

== matlab function CanardUAV_Flight_Control_Using_PID/QUADROTOR /MATLAB Function ==
  data: THETA output; PHI output; T2 input; T3 input; T4 input; PSI output
function [THETA,PHI,PSI] = fcn(T2,T3,T4)
Ix=2.2e-3;
Iy=2.9e-3;
Iz=5.3e-3;

THETA=1.5*T2/Ix; % Pitch
PHI=1.5*T3/Iy;   % Roll
PSI=1.5*T4/Iz;   % Yaw

== matlab function CanardUAV_Flight_Control_Using_PID/QUADROTOR /MATLAB Function1 ==
  data: T input; theta input; phi input; X output; Y output; Z output
function [X,Y,Z] = fcn(T,theta,phi)
g=9.8;
m=0.460;
X=1.5*theta*g;
Y=-1.5*phi*g;
Z=1.5*(1/m)*(T-m*g);
